simulink model "P98_4_1"  (R2016a)
settings: Solver=VariableStepAuto  StartTime=0.0  StopTime=10.0  RelTol=1e-3
settings Model: Creator=Shinelon  LastModifiedBy=Shinelon

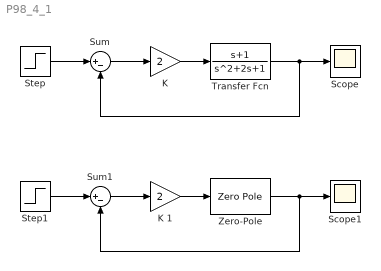
== system P98_4_1 ==
  "K " : Gain  Gain=2
  K 1 : Gain  Gain=2
  Scope : Scope
  Scope1 : Scope
  Step : Step  Time=0  SampleTime=0
  Step1 : Step  Time=0  SampleTime=0
  Sum : Sum  Inputs=|+-
  Sum1 : Sum  Inputs=|+-
  Transfer Fcn : TransferFcn  Numerator=[1 1]
  Zero-Pole : ZeroPole  Zeros=[-1]  Poles=[-1 -1]
  wires:
  Step/1 -> Sum/1
  Sum/1 -> "K "/1
  "K "/1 -> Transfer Fcn/1
  Transfer Fcn/1 -> Sum/2, Scope/1
  Step1/1 -> Sum1/1
  Sum1/1 -> K 1/1
  K 1/1 -> Zero-Pole/1
  Zero-Pole/1 -> Scope1/1, Sum1/2
